simulink model "allModes2"  (R2019a)
settings: Solver=FixedStepAuto  StartTime=0.0  StopTime=inf  FixedStep=1/1000  RelTol=1e-3  EnableMultiTasking=on
undefined symbols (not defined in the file or in its folder): A0, A1, D0, D1, D10, D11, D12, D13, D2, D3, D4, D5, D6, D7, D8, D9, PTA0, PTA1, PTA2, PTB2, PTB23, PTB3, PTB9, PTC16, PTC17, PTC2, PTC3, PTC4, PTD0, PTD1, PTD2, PTD3
libraries: frdmk64flib x22, etargetslib x21, dspstat3 x2
settings Model: SimulationMode=accelerator  ExtModeTrigDuration=5  OrderedModelArguments=off  Creator=adrso  LastModifiedBy=abhis
settings OptimizationCC: EnhancedBackFolding=on  PassReuseOutputArgsAs=Individual arguments  MaxStackSize=64  OptimizeBlockOrder=speed  DifferentSizesBufferReuse=on  OptimizationCustomize=off
settings DebuggingCC: ParameterTunabilityLossMsg=error
settings HardwareCC: ProdBitPerPointer=32  ProdBitPerSizeT=32  ProdBitPerPtrDiffT=32  ProdLargestAtomicInteger=Long  ProdLargestAtomicFloat=Double  ProdWordSize=32  ProdHWDeviceType=ARM Compatible->ARM Cortex
settings SFSimCC: MATLABDynamicMemAlloc=off
settings RTWCC: SystemTargetFile=ert.tlc  HardwareBoard=NXP FRDM-K64F  TLCOptions="-aInlineSetEventsForThisBaseRateFcn=TLC_FALSE -aSuppressMultiTaskScheduler=TLC_FALSE  -aRateBasedStepFcn=0"  TemplateMakefile=ert_default_tmf  GenerateReport=on  Toolchain=GNU Tools for ARM Embedded Processors  BuildConfiguration=Faster Runs  IncludeHyperlinkInReport=on  LaunchReport=on  GenerateTraceInfo=on  GenerateTraceReport=on  GenerateTraceReportSl=on  GenerateTraceReportSf=on  GenerateTraceReportEml=on
settings CodeAppCC: ForceParamTrailComments=on  IgnoreCustomStorageClasses=off  OperatorAnnotations=on  SimulinkDataObjDesc=on  SFDataObjDesc=on  InsertBlockDesc=on
settings ERTTargetCC: SupportContinuousTime=on

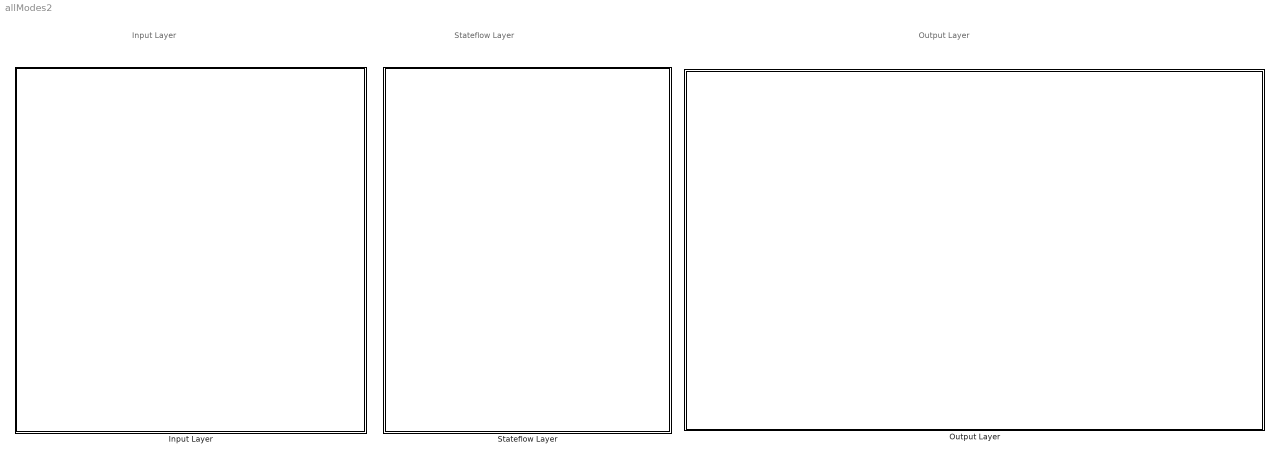
== system allModes2 ==
  note: Input Layer
  note: Stateflow Layer
  note: Output Layer
  Input Layer : Subsystem
      mask Display: image('pacemakerInChest.jpg');
  Output Layer : Subsystem
      mask Display: image('frdmk64f.jpg');
  Stateflow Layer : Subsystem
      mask Display: image('matlabMeme.png');

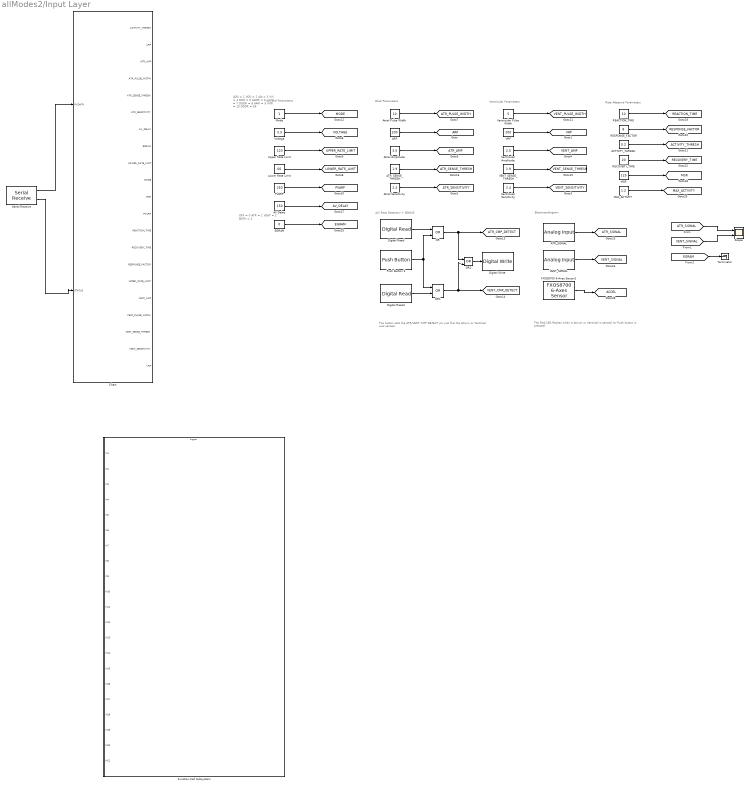
== system allModes2/Input Layer ==
  note: Electrocardiogram
  note: Rate Adaptive Parameters
  note: AOO = 1
      | VOO = 2
      | AAI = 3
      | VVI = 4
      | DOO = 5
      | AOOR = 6
      | VOOR = 7
      | DOOR = 8
      | AAIR = 9
      | VVIR = 10
      | DDDR = 69
  note: The Red LED flashes when a Atrium or Ventrical
      | is sensed (or Push button is pressed)
  note: The button sets the ATR/VENT CMP DETECT
      | pin just like the Atrium or Ventrical was sensed
  note: Ventricular Parameters
  note: Atrial Parameters
  note: A/V Pace Detection + BONUS
  note: General Parameters
  note: OFF = 0
      | ATR = 1
      | VENT = 2
      | BOTH = 3
  ACTIVITY_THRESH : Constant  Value=0.2  OutDataTypeStr=double
  ARP : Constant  Value=200  OutDataTypeStr=uint16
  ATR_SENSE_THRESH : Constant  Value=1.9  OutDataTypeStr=double
  ATR_SIGNAL : frdmk64flib/Analog Input  Whichpin=PTB2 (A0)  SampleTime=-1
      settings: SourceProductName=Simulink Coder Support Package for NXP FRDM-K64F Board
  AV Delay : Constant  Value=150  OutDataTypeStr=uint16
  Atrial Amplitude : Constant  Value=3.5  OutDataTypeStr=double
  Atrial Pulse Width : Constant  Value=10  OutDataTypeStr=uint16
  Atrial Sensitivity : Constant  Value=2.4  OutDataTypeStr=double
  Chart : Stateflow chart  BlockKeywords=__PRM__SERIALIZED__DATA__:Stateflow Chart,Stateflow Diagram  TreatAsAtomicUnit=on
  Digital Read : frdmk64flib/Digital Read  Whichpin=PTC16 (D0)  SampleTime=-1
      settings: SourceProductName=Simulink Coder Support Package for NXP FRDM-K64F Board
  Digital Read1 : frdmk64flib/Digital Read  Whichpin=PTC17 (D1)  SampleTime=-1
      settings: SourceProductName=Simulink Coder Support Package for NXP FRDM-K64F Board
  Digital Write : frdmk64flib/Digital Write  Whichpin=RED_LED
      settings: SourceProductName=Simulink Coder Support Package for NXP FRDM-K64F Board
  EGRAM : Constant  Value=0  OutDataTypeStr=uint16
  FXOS8700 6-Axes Sensor1 : frdmk64flib/FXOS8700 6-Axes Sensor  Activesensor=Accelerometer only  ODR=100Hz  HybridODR=400Hz  Accelfullrange=-4g to +4g  SampleTime=1/100
      settings: SourceProductName=Simulink Coder Support Package for NXP FRDM-K64F Board
  Function-Call Subsystem : Subsystem  TreatAsAtomicUnit=on
  Lower Rate Limit : Constant  Value=60  OutDataTypeStr=uint16
  MAX_ACTIVITY : Constant  Value=1.2  OutDataTypeStr=double
  MSR : Constant  Value=125  OutDataTypeStr=uint16
  Mode : Constant  OutDataTypeStr=uint8
  OR : Logic  Operator=OR  IconShape=distinctive  AllPortsSameDT=off  OutDataTypeStr=boolean
  OR1 : Logic  Operator=OR  IconShape=distinctive  AllPortsSameDT=off  OutDataTypeStr=boolean
  OR2 : Logic  Operator=OR  IconShape=distinctive  AllPortsSameDT=off  OutDataTypeStr=boolean
  PVARP : Constant  Value=250  OutDataTypeStr=uint16
  Push Button 3 : frdmk64flib/Push Button  Whichswitch=SW3  SampleTime1=-1
      settings: SourceProductName=Simulink Coder Support Package for NXP FRDM-K64F Board
  "REACTION_TIME " : Constant  Value=10  OutDataTypeStr=uint16
  RECOVERY_TIME : Constant  Value=20  OutDataTypeStr=uint16
  RESPONSE_FACTOR : Constant  Value=8  OutDataTypeStr=uint16
  Scope : Scope  NumInputPorts=2
  Serial Receive : frdmk64flib/Serial Receive  SCIModule=0  Baudrate=uint32(9600)  Parity=None  StopBits=1  HardwareFlowControl=None  ByteOrder=LittleEndian  DataType=uint8  DataLength=87  BlockingMode=off  OutputStatus=on  SampleTime=-1
      settings: SourceProductName=Simulink Coder Support Package for NXP FRDM-K64F Board
  Terminator : Terminator
  Upper Rate Limit : Constant  Value=120  OutDataTypeStr=uint16
  VENT_SENSE_THRESH : Constant  Value=1.9  OutDataTypeStr=double
  VENT_SIGNAL : frdmk64flib/Analog Input  Whichpin=PTB3 (A1)  SampleTime=-1
      settings: SourceProductName=Simulink Coder Support Package for NXP FRDM-K64F Board
  VRP : Constant  Value=200  OutDataTypeStr=uint16
  Ventricular Amplitude : Constant  Value=2.5  OutDataTypeStr=double
  Ventricular Pulse Width : Constant  Value=5  OutDataTypeStr=uint16
  Ventricular Sensitivity : Constant  Value=2.4  OutDataTypeStr=double
  Voltage : Constant  Value=3.3  OutDataTypeStr=double
  tag scope: ACCEL=global, ACTIVITY_THRESH=global, ARP=global, ATR_AMP=global, ATR_CMP_DETECT=global, ATR_PULSE_WIDTH=global, ATR_SENSE_THRESH=global, ATR_SENSITIVITY=global, ATR_SIGNAL=global, AV_DELAY=global, EGRAM=global, LOWER_RATE_LIMIT=global, MAX_ACTIVITY=global, MODE=global, MSR=global, PVARP=global, REACTION_TIME=global, RECOVERY_TIME=global, RESPONSE_FACTOR=global, UPPER_RATE_LIMIT=global, VENT_AMP=global, VENT_CMP_DETECT=global, VENT_PULSE_WIDTH=global, VENT_SENSE_THRESH=global, VENT_SENSITIVITY=global, VENT_SIGNAL=global, VOLTAGE=global, VRP=global
  wires:
  Ventricular Amplitude/1 -> [VENT_AMP]
  ARP/1 -> [ARP]
  Atrial Amplitude/1 -> [ATR_AMP]
  VRP/1 -> [VRP]
  Voltage/1 -> [VOLTAGE]
  Atrial Sensitivity/1 -> [ATR_SENSITIVITY]
  Ventricular Sensitivity/1 -> [VENT_SENSITIVITY]
  Upper Rate Limit/1 -> [UPPER_RATE_LIMIT]
  Mode/1 -> [MODE]
  Lower Rate Limit/1 -> [LOWER_RATE_LIMIT]
  Ventricular Pulse Width/1 -> [VENT_PULSE_WIDTH]
  Atrial Pulse Width/1 -> [ATR_PULSE_WIDTH]
  Digital Read1/1 -> OR1/2
  VENT_SENSE_THRESH/1 -> [VENT_SENSE_THRESH]
  ATR_SENSE_THRESH/1 -> [ATR_SENSE_THRESH]
  OR/1 -> OR2/1, [ATR_CMP_DETECT]
  Digital Read/1 -> OR/1
  Push Button 3/1 -> OR/2, OR1/1
  OR1/1 -> OR2/2, [VENT_CMP_DETECT]
  OR2/1 -> Digital Write/1
  PVARP/1 -> [PVARP]
  AV Delay/1 -> [AV_DELAY]
  "REACTION_TIME "/1 -> [REACTION_TIME]
  RESPONSE_FACTOR/1 -> [RESPONSE_FACTOR]
  ACTIVITY_THRESH/1 -> [ACTIVITY_THRESH]
  RECOVERY_TIME/1 -> [RECOVERY_TIME]
  MSR/1 -> [MSR]
  ATR_SIGNAL/1 -> [ATR_SIGNAL]
  VENT_SIGNAL/1 -> [VENT_SIGNAL]
  [VENT_SIGNAL] -> Scope/2
  [ATR_SIGNAL] -> Scope/1
  EGRAM/1 -> [EGRAM]
  [EGRAM] -> Terminator/1
  MAX_ACTIVITY/1 -> [MAX_ACTIVITY]
  FXOS8700 6-Axes Sensor1/1 -> [ACCEL]
  Serial Receive/2 -> Chart/2(STATUS)
  Serial Receive/1 -> Chart/1(RXDATA)

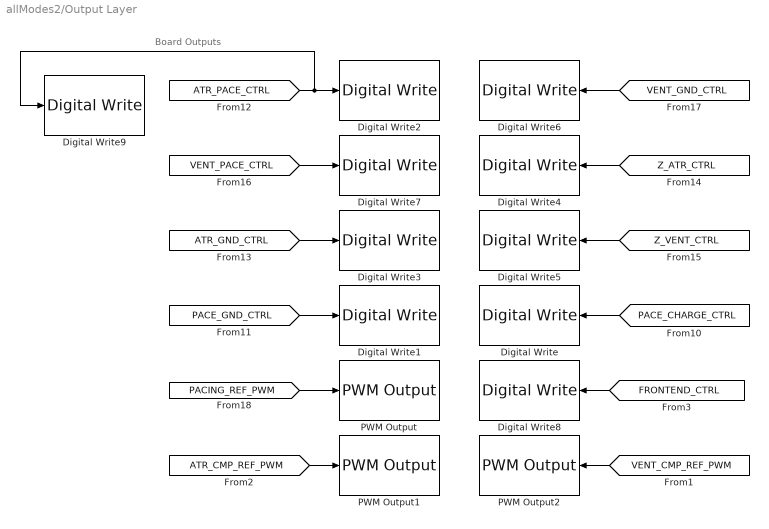
== system allModes2/Output Layer ==
  note: Board Outputs
  Digital Write : frdmk64flib/Digital Write  Whichpin=PTB9 (D2)
      settings: SourceProductName=Simulink Coder Support Package for NXP FRDM-K64F Board
  Digital Write1 : frdmk64flib/Digital Write  Whichpin=PTD0 (D10)
      settings: SourceProductName=Simulink Coder Support Package for NXP FRDM-K64F Board
  Digital Write2 : frdmk64flib/Digital Write  Whichpin=PTA0 (D8)
      settings: SourceProductName=Simulink Coder Support Package for NXP FRDM-K64F Board
  Digital Write3 : frdmk64flib/Digital Write  Whichpin=PTD2 (D11)
      settings: SourceProductName=Simulink Coder Support Package for NXP FRDM-K64F Board
  Digital Write4 : frdmk64flib/Digital Write  Whichpin=PTB23 (D4)
      settings: SourceProductName=Simulink Coder Support Package for NXP FRDM-K64F Board
  Digital Write5 : frdmk64flib/Digital Write  Whichpin=PTC3 (D7)
      settings: SourceProductName=Simulink Coder Support Package for NXP FRDM-K64F Board
  Digital Write6 : frdmk64flib/Digital Write  Whichpin=PTD3 (D12)
      settings: SourceProductName=Simulink Coder Support Package for NXP FRDM-K64F Board
  Digital Write7 : frdmk64flib/Digital Write  Whichpin=PTC4 (D9)
      settings: SourceProductName=Simulink Coder Support Package for NXP FRDM-K64F Board
  Digital Write8 : frdmk64flib/Digital Write  Whichpin=PTD1 (D13)
      settings: SourceProductName=Simulink Coder Support Package for NXP FRDM-K64F Board
  Digital Write9 : frdmk64flib/Digital Write  Whichpin=GREEN_LED
      settings: SourceProductName=Simulink Coder Support Package for NXP FRDM-K64F Board
  PWM Output : frdmk64flib/PWM Output  Whichpin=PTA2 (D5)  InitialFrequency=2000  InitialDutyCycle=30
      settings: SourceProductName=Simulink Coder Support Package for NXP FRDM-K64F Board
  PWM Output1 : frdmk64flib/PWM Output  Whichpin=PTC2 (D6)  InitialFrequency=2000  InitialDutyCycle=30
      settings: SourceProductName=Simulink Coder Support Package for NXP FRDM-K64F Board
  PWM Output2 : frdmk64flib/PWM Output  Whichpin=PTA1 (D3)  InitialFrequency=2000  InitialDutyCycle=30
      settings: SourceProductName=Simulink Coder Support Package for NXP FRDM-K64F Board
  wires:
  [PACING_REF_PWM] -> PWM Output/1
  [VENT_GND_CTRL] -> Digital Write6/1
  [ATR_GND_CTRL] -> Digital Write3/1
  [VENT_PACE_CTRL] -> Digital Write7/1
  [PACE_CHARGE_CTRL] -> Digital Write/1
  [ATR_PACE_CTRL] -> Digital Write9/1, Digital Write2/1
  [Z_VENT_CTRL] -> Digital Write5/1
  [Z_ATR_CTRL] -> Digital Write4/1
  [PACE_GND_CTRL] -> Digital Write1/1
  [ATR_CMP_REF_PWM] -> PWM Output1/1
  [VENT_CMP_REF_PWM] -> PWM Output2/1
  [FRONTEND_CTRL] -> Digital Write8/1

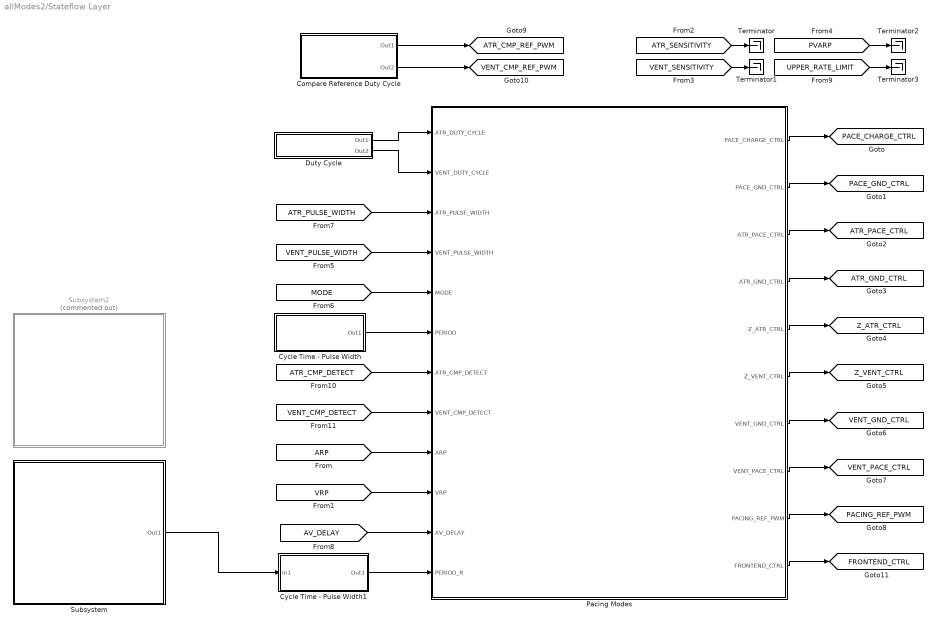
== system allModes2/Stateflow Layer ==
  Compare Reference Duty Cycle : Subsystem
  Cycle Time - Pulse Width : Subsystem
  Cycle Time - Pulse Width1 : Subsystem
  Duty Cycle : Subsystem
  Pacing Modes : Stateflow chart  BlockKeywords=__PRM__SERIALIZED__DATA__:Stateflow Chart,Stateflow Diagram  TreatAsAtomicUnit=on
  Subsystem : Subsystem
  Subsystem2 : Subsystem  Commented=on
  Terminator{,1..3} (4 alike) : Terminator
  tag scope: ATR_CMP_REF_PWM=global, ATR_GND_CTRL=global, ATR_PACE_CTRL=global, FRONTEND_CTRL=global, PACE_CHARGE_CTRL=global, PACE_GND_CTRL=global, PACING_REF_PWM=global, VENT_CMP_REF_PWM=global, VENT_GND_CTRL=global, VENT_PACE_CTRL=global, Z_ATR_CTRL=global, Z_VENT_CTRL=global
  wires:
  [ATR_PULSE_WIDTH] -> Pacing Modes/3(ATR_PULSE_WIDTH)
  [VENT_PULSE_WIDTH] -> Pacing Modes/4(VENT_PULSE_WIDTH)
  Duty Cycle/1(Out1) -> Pacing Modes/1(ATR_DUTY_CYCLE)
  Duty Cycle/2(Out2) -> Pacing Modes/2(VENT_DUTY_CYCLE)
  Pacing Modes/6(Z_VENT_CTRL) -> [Z_VENT_CTRL]
  Pacing Modes/8(VENT_PACE_CTRL) -> [VENT_PACE_CTRL]
  Pacing Modes/4(ATR_GND_CTRL) -> [ATR_GND_CTRL]
  Pacing Modes/3(ATR_PACE_CTRL) -> [ATR_PACE_CTRL]
  Pacing Modes/9(PACING_REF_PWM) -> [PACING_REF_PWM]
  Pacing Modes/2(PACE_GND_CTRL) -> [PACE_GND_CTRL]
  Pacing Modes/1(PACE_CHARGE_CTRL) -> [PACE_CHARGE_CTRL]
  Pacing Modes/5(Z_ATR_CTRL) -> [Z_ATR_CTRL]
  Pacing Modes/7(VENT_GND_CTRL) -> [VENT_GND_CTRL]
  [MODE] -> Pacing Modes/5(MODE)
  Cycle Time - Pulse Width/1(Out1) -> Pacing Modes/6(PERIOD)
  [VENT_CMP_DETECT] -> Pacing Modes/8(VENT_CMP_DETECT)
  [ATR_CMP_DETECT] -> Pacing Modes/7(ATR_CMP_DETECT)
  Pacing Modes/10(FRONTEND_CTRL) -> [FRONTEND_CTRL]
  [ARP] -> Pacing Modes/9(ARP)
  [VRP] -> Pacing Modes/10(VRP)
  Compare Reference Duty Cycle/1(Out1) -> [ATR_CMP_REF_PWM]
  Compare Reference Duty Cycle/2(Out2) -> [VENT_CMP_REF_PWM]
  [ATR_SENSITIVITY] -> Terminator/1
  [VENT_SENSITIVITY] -> Terminator1/1
  [UPPER_RATE_LIMIT] -> Terminator3/1
  [PVARP] -> Terminator2/1
  [AV_DELAY] -> Pacing Modes/11(AV_DELAY)
  Cycle Time - Pulse Width1/1(Out1) -> Pacing Modes/12(PERIOD_R)
  Subsystem/1(Out1) -> Cycle Time - Pulse Width1/1(In1)

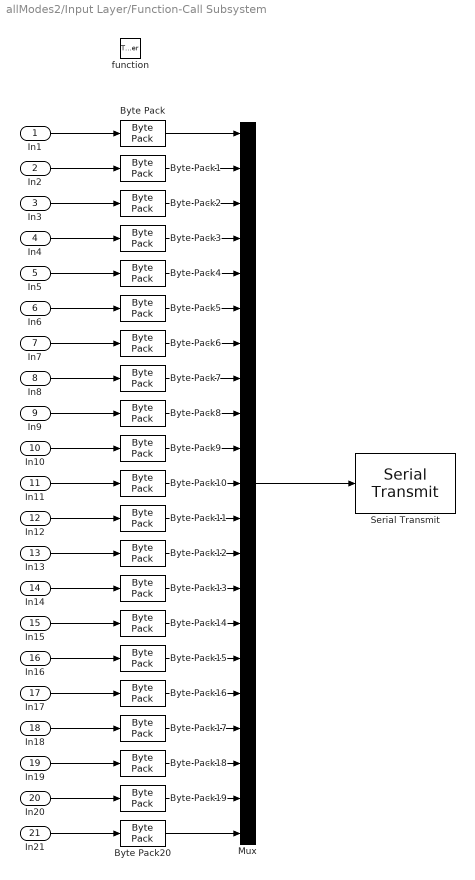
== system allModes2/Input Layer/Function-Call Subsystem ==
  In1 : Inport
  In2 : Inport  Port=2
  In3 : Inport  Port=3
  In4 : Inport  Port=4
  In5 : Inport  Port=5
  In6 : Inport  Port=6
  In7 : Inport  Port=7
  In8 : Inport  Port=8
  In9 : Inport  Port=9
  In10 : Inport  Port=10
  In11 : Inport  Port=11
  In12 : Inport  Port=12
  In13 : Inport  Port=13
  In14 : Inport  Port=14
  In15 : Inport  Port=15
  In16 : Inport  Port=16
  In17 : Inport  Port=17
  In18 : Inport  Port=18
  In19 : Inport  Port=19
  In20 : Inport  Port=20
  In21 : Inport  Port=21
  function : TriggerPort  TriggerType=function-call  IsSimulinkFunction=on  FunctionName=SEND_PARAMETERS  VariantControl=Variant
  Byte Pack{,1..20} (21 alike) : etargetslib/Byte Pack  datatypes={'double'}  byteAlign=1
      settings: SourceProductName=MATLAB Coder
  Mux : Mux  Inputs=21
  Serial Transmit : frdmk64flib/Serial Transmit  SCIModule=0  Baudrate=uint32(9600)  Parity=None  StopBits=1  HardwareFlowControl=None  ByteOrder=LittleEndian  BlockingMode=on  OutputStatus=off
      settings: SourceProductName=Simulink Coder Support Package for NXP FRDM-K64F Board
  wires:
  In1/1 -> Byte Pack/1
  In2/1 -> Byte Pack1/1
  In3/1 -> Byte Pack2/1
  In4/1 -> Byte Pack3/1
  In5/1 -> Byte Pack4/1
  In6/1 -> Byte Pack5/1
  In7/1 -> Byte Pack6/1
  In8/1 -> Byte Pack7/1
  In9/1 -> Byte Pack8/1
  In10/1 -> Byte Pack9/1
  In11/1 -> Byte Pack10/1
  In12/1 -> Byte Pack11/1
  In13/1 -> Byte Pack12/1
  In14/1 -> Byte Pack13/1
  In15/1 -> Byte Pack14/1
  In16/1 -> Byte Pack15/1
  In17/1 -> Byte Pack16/1
  In18/1 -> Byte Pack17/1
  In19/1 -> Byte Pack18/1
  In20/1 -> Byte Pack19/1
  In21/1 -> Byte Pack20/1
  Byte Pack/1 -> Mux/1
  Byte Pack1/1 -> Mux/2
  Byte Pack2/1 -> Mux/3
  Byte Pack3/1 -> Mux/4
  Byte Pack4/1 -> Mux/5
  Byte Pack5/1 -> Mux/6
  Byte Pack6/1 -> Mux/7
  Byte Pack7/1 -> Mux/8
  Byte Pack8/1 -> Mux/9
  Byte Pack9/1 -> Mux/10
  Byte Pack10/1 -> Mux/11
  Byte Pack11/1 -> Mux/12
  Byte Pack12/1 -> Mux/13
  Byte Pack13/1 -> Mux/14
  Byte Pack14/1 -> Mux/15
  Byte Pack15/1 -> Mux/16
  Byte Pack16/1 -> Mux/17
  Byte Pack17/1 -> Mux/18
  Byte Pack18/1 -> Mux/19
  Byte Pack19/1 -> Mux/20
  Byte Pack20/1 -> Mux/21
  Mux/1 -> Serial Transmit/1

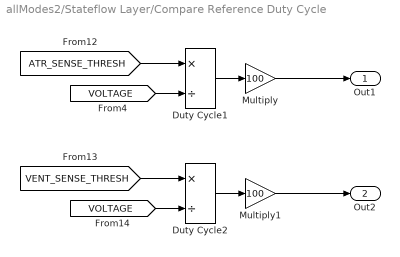
== system allModes2/Stateflow Layer/Compare Reference Duty Cycle ==
  Duty Cycle1 : Product  Inputs=*/
  Duty Cycle2 : Product  Inputs=*/
  Multiply : Gain  Gain=100
  Multiply1 : Gain  Gain=100
  Out1 : Outport
  Out2 : Outport  Port=2
  wires:
  Multiply1/1 -> Out2/1
  [VENT_SENSE_THRESH] -> Duty Cycle2/1
  [VOLTAGE] -> Duty Cycle1/2
  [VOLTAGE] -> Duty Cycle2/2
  Duty Cycle2/1 -> Multiply1/1
  [ATR_SENSE_THRESH] -> Duty Cycle1/1
  Duty Cycle1/1 -> Multiply/1
  Multiply/1 -> Out1/1

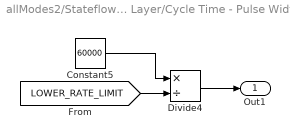
== system allModes2/Stateflow Layer/Cycle Time - Pulse Width ==
  Constant5 : Constant  Value=60000  OutDataTypeStr=uint16
  Divide4 : Product  Inputs=*/  OutDataTypeStr=uint16  RndMeth=Nearest
  Out1 : Outport
  wires:
  [LOWER_RATE_LIMIT] -> Divide4/2
  Constant5/1 -> Divide4/1
  Divide4/1 -> Out1/1

== system allModes2/Stateflow Layer/Cycle Time - Pulse Width1 ==
  In1 : Inport
  Constant5 : Constant  Value=60000  OutDataTypeStr=uint16
  Divide4 : Product  Inputs=*/  OutDataTypeStr=uint16  RndMeth=Nearest
  Out1 : Outport
  wires:
  Constant5/1 -> Divide4/1
  In1/1 -> Divide4/2
  Divide4/1 -> Out1/1

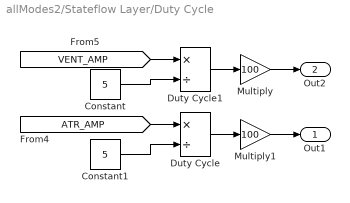
== system allModes2/Stateflow Layer/Duty Cycle ==
  Constant : Constant  Value=5
  Constant1 : Constant  Value=5
  Duty Cycle : Product  Inputs=*/
  Duty Cycle1 : Product  Inputs=*/
  Multiply : Gain  Gain=100
  Multiply1 : Gain  Gain=100
  Out1 : Outport
  Out2 : Outport  Port=2
  wires:
  Constant1/1 -> Duty Cycle/2
  [ATR_AMP] -> Duty Cycle/1
  Constant/1 -> Duty Cycle1/2
  [VENT_AMP] -> Duty Cycle1/1
  Duty Cycle1/1 -> Multiply/1
  Multiply/1 -> Out2/1
  Multiply1/1 -> Out1/1
  Duty Cycle/1 -> Multiply1/1

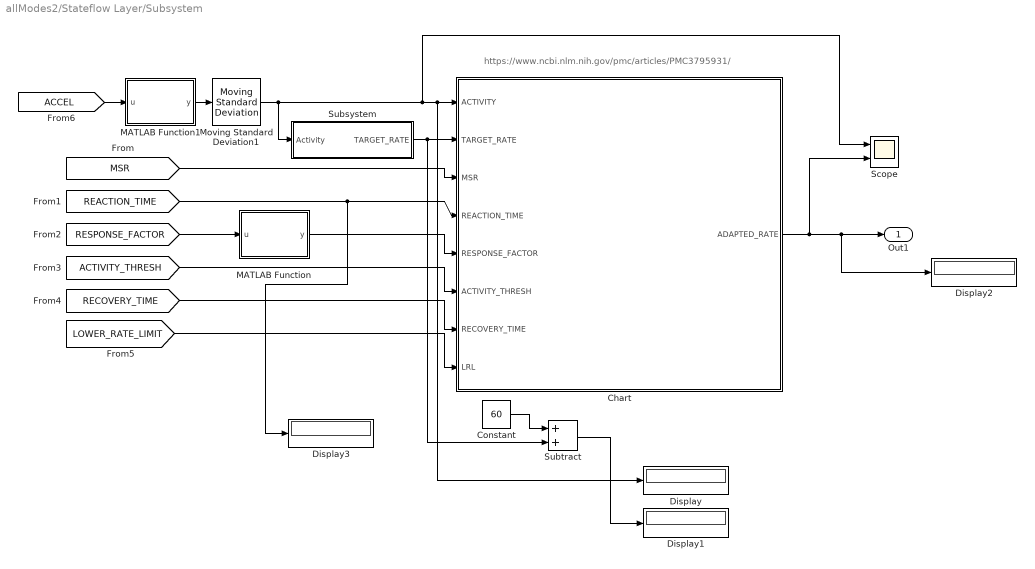
== system allModes2/Stateflow Layer/Subsystem ==
  note: https://www.ncbi.nlm.nih.gov/pmc/articles/PMC3795931/
  Chart : Stateflow chart  BlockKeywords=__PRM__SERIALIZED__DATA__:Stateflow Chart,Stateflow Diagram  TreatAsAtomicUnit=on
  Constant : Constant  Value=60
  Display{,1..3} (4 alike) : Display
  MATLAB Function : MATLAB Function  TreatAsAtomicUnit=on
  MATLAB Function1 : MATLAB Function  TreatAsAtomicUnit=on
  Moving Standard Deviation1 : dspstat3/Moving Standard Deviation  Method=Sliding window  ForgettingFactorPort=off  SpecifyWindowLength=on  WindowLength=64  ForgettingFactor=0.9  SimulateUsing=Code generation
      settings: SourceProductName=DSP System Toolbox  SourceProductBaseCode=DS
  Scope : Scope  NumInputPorts=2
  Subsystem : Subsystem
  Subtract : Sum
  Out1 : Outport
  wires:
  [ACCEL] -> MATLAB Function1/1(u)
  MATLAB Function1/1(y) -> Moving Standard Deviation1/1
  Moving Standard Deviation1/1 -> Scope/1, Display/1, Chart/1(ACTIVITY), Subsystem/1(Activity)
  [MSR] -> Chart/3(MSR)
  [REACTION_TIME] -> Display3/1, Chart/4(REACTION_TIME)
  [ACTIVITY_THRESH] -> Chart/6(ACTIVITY_THRESH)
  [RECOVERY_TIME] -> Chart/7(RECOVERY_TIME)
  [LOWER_RATE_LIMIT] -> Chart/8(LRL)
  Subsystem/1(TARGET_RATE) -> Subtract/2, Chart/2(TARGET_RATE)
  [RESPONSE_FACTOR] -> MATLAB Function/1(u)
  MATLAB Function/1(y) -> Chart/5(RESPONSE_FACTOR)
  Chart/1(ADAPTED_RATE) -> Display2/1, Out1/1, Scope/2
  Constant/1 -> Subtract/1
  Subtract/1 -> Display1/1

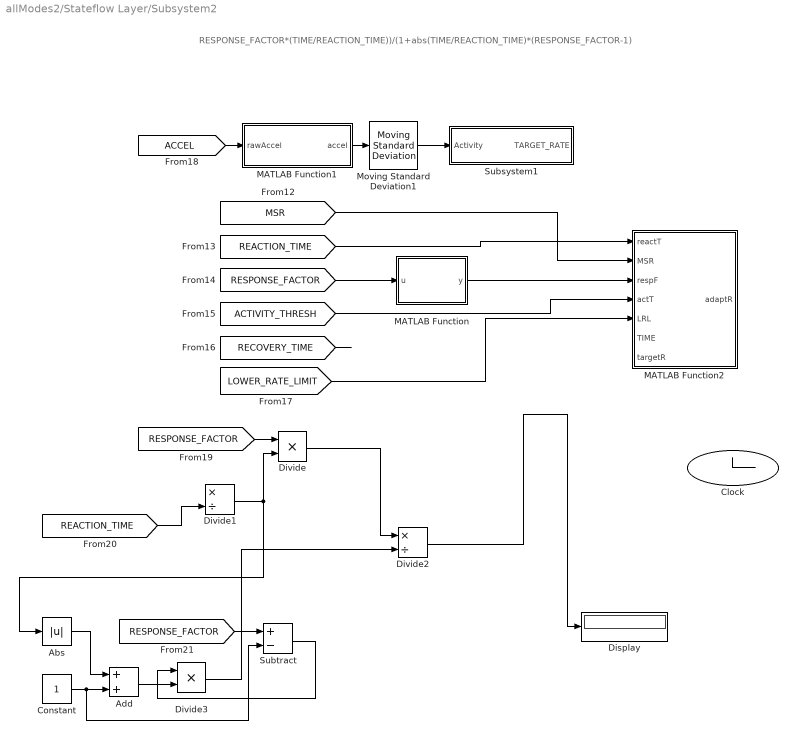
== system allModes2/Stateflow Layer/Subsystem2 ==
  note: RESPONSE_FACTOR*(TIME/REACTION_TIME))/(1+abs(TIME/REACTION_TIME)*(RESPONSE_FACTOR-1)
  Abs : Abs
  Add : Sum
  Clock : Clock
      settings: Decimation=1000
  Constant : Constant
  Display : Display
  Divide : Product  Inputs=**
  Divide1 : Product  Inputs=*/
  Divide2 : Product  Inputs=*/
  Divide3 : Product  Inputs=**
  MATLAB Function : MATLAB Function  TreatAsAtomicUnit=on
  MATLAB Function1 : MATLAB Function  TreatAsAtomicUnit=on
  MATLAB Function2 : MATLAB Function  TreatAsAtomicUnit=on
  Moving Standard Deviation1 : dspstat3/Moving Standard Deviation  Method=Sliding window  ForgettingFactorPort=off  SpecifyWindowLength=on  WindowLength=600  ForgettingFactor=0.9  SimulateUsing=Code generation
      settings: SourceProductName=DSP System Toolbox  SourceProductBaseCode=DS
  Subsystem1 : Subsystem
  Subtract : Sum  Inputs=+-
  wires:
  Divide2/1 -> Display/1
  [RESPONSE_FACTOR] -> Divide/1
  [RESPONSE_FACTOR] -> Subtract/1
  Abs/1 -> Add/1
  Constant/1 -> Subtract/2, Add/2
  Add/1 -> Divide3/2
  Moving Standard Deviation1/1 -> Subsystem1/1(Activity)
  Divide/1 -> Divide2/1
  ? -> Divide1/1
  [RESPONSE_FACTOR] -> MATLAB Function/1(u)
  MATLAB Function1/1(accel) -> Moving Standard Deviation1/1
  [REACTION_TIME] -> Divide1/2
  [ACCEL] -> MATLAB Function1/1(rawAccel)
  Subtract/1 -> Divide3/1
  Divide1/1 -> Abs/1, Divide/2
  Divide3/1 -> Divide2/2
  MATLAB Function/1(y) -> MATLAB Function2/3(respF)
  [REACTION_TIME] -> MATLAB Function2/1(reactT)
  [MSR] -> MATLAB Function2/2(MSR)
  [ACTIVITY_THRESH] -> MATLAB Function2/4(actT)
  [LOWER_RATE_LIMIT] -> MATLAB Function2/5(LRL)
  [RECOVERY_TIME] -> ?

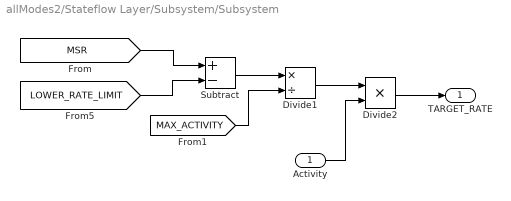
== system allModes2/Stateflow Layer/Subsystem/Subsystem ==
  Activity : Inport
  Divide1 : Product  Inputs=*/
  Divide2 : Product  Inputs=**  OutDataTypeStr=uint16  RndMeth=Nearest
  Subtract : Sum  Inputs=+-
  TARGET_RATE : Outport
  wires:
  [MSR] -> Subtract/1
  [LOWER_RATE_LIMIT] -> Subtract/2
  Subtract/1 -> Divide1/1
  Divide1/1 -> Divide2/1
  Activity/1 -> Divide2/2
  Divide2/1 -> TARGET_RATE/1
  [MAX_ACTIVITY] -> Divide1/2

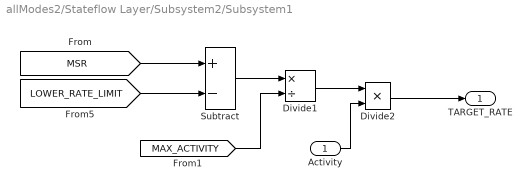
== system allModes2/Stateflow Layer/Subsystem2/Subsystem1 ==
  Activity : Inport
  Divide1 : Product  Inputs=*/
  Divide2 : Product  Inputs=**  OutDataTypeStr=uint16
  Subtract : Sum  Inputs=+-
  TARGET_RATE : Outport
  wires:
  [MSR] -> Subtract/1
  [LOWER_RATE_LIMIT] -> Subtract/2
  Subtract/1 -> Divide1/1
  Divide1/1 -> Divide2/1
  Activity/1 -> Divide2/2
  Divide2/1 -> TARGET_RATE/1
  [MAX_ACTIVITY] -> Divide1/2

== matlab function allModes2/Stateflow Layer/Subsystem/MATLAB Function1 ==
  data: u input; y output
function y = fcn(u)
y = sqrt(u(1)^2+u(2)^2+u(3)^2);

== stateflow chart allModes2/Stateflow Layer/Subsystem/Chart ==
  state Up
    entry:
    TIME = 0
    during:
    ADAPTED_RATE = RESPONSE_FACTOR*(TIME/10)/(1+abs(TIME/10)*(RESPONSE_FACTOR-1))*TARGET_RATE + LRL
    TIME = TIME + 1/1000
    exit:
    TIME = 0
  state Max
  state Down
    entry:
    TIME = 0
    DELTA_RATE = ADAPTED_RATE - LRL
    during:
    ADAPTED_RATE = ADAPTED_RATE - (DELTA_RATE/RECOVERY_TIME)*TIME
    TIME = TIME + 1/1000
    exit:
    TIME = 0
  state Start
    entry:
    ADAPTED_RATE = LRL
  state Min
  Up -> Up [order 3] : [TIME >= REACTION_TIME]{TIME = 0}
  Up -> Max [order 1] : [ADAPTED_RATE == MSR]
  Min -> Up : [ACTIVITY >= ACTIVITY_THRESH]
  Max -> Down : [ACTIVITY < ACTIVITY_THRESH]
  Up -> Down [order 2] : [ACTIVITY < ACTIVITY_THRESH]
  Down -> Up [order 3] : [ACTIVITY >= ACTIVITY_THRESH]
  (default) -> Start
  Start -> Down
  Down -> Min [order 1] : [ADAPTED_RATE == LRL]
  Down -> Down [order 2] : [TIME >= RECOVERY_TIME]{TIME = 0}
  data: ACTIVITY input double; TARGET_RATE input; ADAPTED_RATE output uint16; MSR input uint16; REACTION_TIME input uint16; RESPONSE_FACTOR input double; ACTIVITY_THRESH input double; RECOVERY_TIME input uint16; LRL input uint16; DELTA_RATE local uint16; TIME local double

== stateflow chart allModes2/Stateflow Layer/Pacing Modes ==
  state DOO [group]
    state ATR_DISCHARGING
      during:
      %Discharge C22 into ATR
      %Charge C21
      PACE_CHARGE_CTRL = false
      PACE_GND_CTRL = true
      ATR_PACE_CTRL = true
      ATR_GND_CTRL = false
      Z_ATR_CTRL = false
      Z_VENT_CTRL = false
      VENT_GND_CTRL = false
      VENT_PACE_CTRL = false
    state VENT_CHARGING
      during:
      %Charge C22
      ATR_PACE_CTRL = false
      VENT_PACE_CTRL = false
      PACING_REF_PWM = VENT_DUTY_CYCLE
      PACE_CHARGE_CTRL = true
      %Discharge C21
      PACE_GND_CTRL = true
      VENT_PACE_CTRL = false
      Z_ATR_CTRL = false
      Z_VENT_CTRL = false
      ATR_PACE_CTRL = false
      ATR_GND_CTRL = true
      VENT_GND_CTRL = false
    state VENT_DISCHARGING
      during:
      %Discharge C22 into VENT
      %Charge C21
      PACE_CHARGE_CTRL = false
      PACE_GND_CTRL = true
      ATR_PACE_CTRL = false
      ATR_GND_CTRL = false
      Z_ATR_CTRL = false
      Z_VENT_CTRL = false
      VENT_GND_CTRL = false
      VENT_PACE_CTRL = true
    state ATR_CHARGING
      during:
      %Charge C22
      ATR_PACE_CTRL = false
      VENT_PACE_CTRL = false
      PACING_REF_PWM = VENT_DUTY_CYCLE
      PACE_CHARGE_CTRL = true
      %Discharge C21
      PACE_GND_CTRL = true
      VENT_PACE_CTRL = false
      Z_ATR_CTRL = false
      Z_VENT_CTRL = false
      ATR_PACE_CTRL = false
      ATR_GND_CTRL = false
      VENT_GND_CTRL = true
    DOO.ATR_DISCHARGING -> DOO.VENT_CHARGING : after(ATR_PULSE_WIDTH,msec)
    DOO.VENT_CHARGING -> DOO.VENT_DISCHARGING : after(AV_DELAY - ATR_PULSE_WIDTH, msec)
    DOO.ATR_CHARGING -> DOO.ATR_DISCHARGING [order 2] : after(PERIOD - VENT_PULSE_WIDTH - AV_DELAY, msec)
    DOO.VENT_DISCHARGING -> DOO.ATR_CHARGING : after(VENT_PULSE_WIDTH,msec)
  state DOOR [group]
    state ATR_DISCHARGING
      during:
      %Discharge C22 into ATR
      %Charge C21
      PACE_CHARGE_CTRL = false
      PACE_GND_CTRL = true
      ATR_PACE_CTRL = true
      ATR_GND_CTRL = false
      Z_ATR_CTRL = false
      Z_VENT_CTRL = false
      VENT_GND_CTRL = false
      VENT_PACE_CTRL = false
    state VENT_CHARGING
      during:
      %Charge C22
      ATR_PACE_CTRL = false
      VENT_PACE_CTRL = false
      PACING_REF_PWM = VENT_DUTY_CYCLE
      PACE_CHARGE_CTRL = true
      %Discharge C21
      PACE_GND_CTRL = true
      VENT_PACE_CTRL = false
      Z_ATR_CTRL = false
      Z_VENT_CTRL = false
      ATR_PACE_CTRL = false
      ATR_GND_CTRL = true
      VENT_GND_CTRL = false
    state VENT_DISCHARGING
      during:
      %Discharge C22 into VENT
      %Charge C21
      PACE_CHARGE_CTRL = false
      PACE_GND_CTRL = true
      ATR_PACE_CTRL = false
      ATR_GND_CTRL = false
      Z_ATR_CTRL = false
      Z_VENT_CTRL = false
      VENT_GND_CTRL = false
      VENT_PACE_CTRL = true
    state ATR_CHARGING
      during:
      %Charge C22
      ATR_PACE_CTRL = false
      VENT_PACE_CTRL = false
      PACING_REF_PWM = VENT_DUTY_CYCLE
      PACE_CHARGE_CTRL = true
      %Discharge C21
      PACE_GND_CTRL = true
      VENT_PACE_CTRL = false
      Z_ATR_CTRL = false
      Z_VENT_CTRL = false
      ATR_PACE_CTRL = false
      ATR_GND_CTRL = false
      VENT_GND_CTRL = true
    DOOR.ATR_DISCHARGING -> DOOR.VENT_CHARGING : after(ATR_PULSE_WIDTH,msec)
    DOOR.VENT_CHARGING -> DOOR.VENT_DISCHARGING : after(AV_DELAY - ATR_PULSE_WIDTH, msec)
    DOOR.ATR_CHARGING -> DOOR.ATR_DISCHARGING [order 1] : after(PERIOD_R - VENT_PULSE_WIDTH - AV_DELAY, msec)
    DOOR.VENT_DISCHARGING -> DOOR.ATR_CHARGING : after(VENT_PULSE_WIDTH,msec)
  state AAIR [group]
    state INTERMIDIATE
      during:
      %Discharge C21
      PACE_GND_CTRL = true
      VENT_PACE_CTRL = false
      Z_ATR_CTRL = false
      Z_VENT_CTRL = false
      ATR_PACE_CTRL = false
      ATR_GND_CTRL = true
      VENT_GND_CTRL = false
      %Charge C22
      ATR_PACE_CTRL = false
      VENT_PACE_CTRL = false
      PACING_REF_PWM = ATR_DUTY_CYCLE
      PACE_CHARGE_CTRL = true
    state CHARGING
      during:
      %Charge C22
      ATR_PACE_CTRL = false
      VENT_PACE_CTRL = false
      PACING_REF_PWM = ATR_DUTY_CYCLE
      PACE_CHARGE_CTRL = true
      %Discharge C21
      PACE_GND_CTRL = true
      VENT_PACE_CTRL = false
      Z_ATR_CTRL = false
      Z_VENT_CTRL = false
      ATR_PACE_CTRL = false
      ATR_GND_CTRL = true
      VENT_GND_CTRL = false
    state DISCHARGING
      during:
      %Discharge C22 into ATR
      %Charge C21
      PACE_CHARGE_CTRL = false
      PACE_GND_CTRL = true
      ATR_PACE_CTRL = true
      ATR_GND_CTRL = false
      Z_ATR_CTRL = false
      Z_VENT_CTRL = false
      VENT_GND_CTRL = false
      VENT_PACE_CTRL = false
    AAIR.CHARGING -> (junction 431) [order 1] : [ATR_CMP_DETECT == true]
    (junction 431) -> AAIR.INTERMIDIATE : after(ATR_PULSE_WIDTH,msec)
    AAIR.DISCHARGING -> AAIR.INTERMIDIATE : after(ATR_PULSE_WIDTH, msec)
    AAIR.INTERMIDIATE -> AAIR.CHARGING : after(ARP, msec)
    AAIR.CHARGING -> AAIR.DISCHARGING [order 2] : after(PERIOD_R - ARP - ATR_PULSE_WIDTH, msec)
  state Start
  state AAI [group]
    state INTERMIDIATE
      during:
      %Discharge C21
      PACE_GND_CTRL = true
      VENT_PACE_CTRL = false
      Z_ATR_CTRL = false
      Z_VENT_CTRL = false
      ATR_PACE_CTRL = false
      ATR_GND_CTRL = true
      VENT_GND_CTRL = false
      %Charge C22
      ATR_PACE_CTRL = false
      VENT_PACE_CTRL = false
      PACING_REF_PWM = ATR_DUTY_CYCLE
      PACE_CHARGE_CTRL = true
    state CHARGING
      during:
      %Charge C22
      ATR_PACE_CTRL = false
      VENT_PACE_CTRL = false
      PACING_REF_PWM = ATR_DUTY_CYCLE
      PACE_CHARGE_CTRL = true
      %Discharge C21
      PACE_GND_CTRL = true
      VENT_PACE_CTRL = false
      Z_ATR_CTRL = false
      Z_VENT_CTRL = false
      ATR_PACE_CTRL = false
      ATR_GND_CTRL = true
      VENT_GND_CTRL = false
    state DISCHARGING
      during:
      %Discharge C22 into ATR
      %Charge C21
      PACE_CHARGE_CTRL = false
      PACE_GND_CTRL = true
      ATR_PACE_CTRL = true
      ATR_GND_CTRL = false
      Z_ATR_CTRL = false
      Z_VENT_CTRL = false
      VENT_GND_CTRL = false
      VENT_PACE_CTRL = false
    AAI.CHARGING -> (junction 352) [order 1] : [ATR_CMP_DETECT == true]
    (junction 352) -> AAI.INTERMIDIATE : after(ATR_PULSE_WIDTH,msec)
    AAI.DISCHARGING -> AAI.INTERMIDIATE : after(ATR_PULSE_WIDTH, msec)
    AAI.INTERMIDIATE -> AAI.CHARGING : after(ARP, msec)
    AAI.CHARGING -> AAI.DISCHARGING [order 2] : after(PERIOD - ARP - ATR_PULSE_WIDTH, msec)
  state AAI1 [group]
    state CHARGING
      during:
      %Charge C22
      ATR_PACE_CTRL = false
      VENT_PACE_CTRL = false
      PACING_REF_PWM = ATR_DUTY_CYCLE
      PACE_CHARGE_CTRL = true
      %Discharge C21
      PACE_GND_CTRL = true
      VENT_PACE_CTRL = false
      Z_ATR_CTRL = false
      Z_VENT_CTRL = false
      ATR_PACE_CTRL = false
      ATR_GND_CTRL = true
      VENT_GND_CTRL = false
    state DISCHARGING
      during:
      %Discharge C22 into ATR
      %Charge C21
      PACE_CHARGE_CTRL = false
      PACE_GND_CTRL = true
      ATR_PACE_CTRL = true
      ATR_GND_CTRL = false
      Z_ATR_CTRL = false
      Z_VENT_CTRL = false
      VENT_GND_CTRL = false
      VENT_PACE_CTRL = false
    state w
    AAI1.DISCHARGING -> AAI1.CHARGING : after(ATR_PULSE_WIDTH, msec)
    (junction 410) -> AAI1.CHARGING : after(ATR_PULSE_WIDTH, msec)
    w -> (junction 410) [order 1] : [ATR_CMP_DETECT == true]
    AAI1.CHARGING -> w [order 1] : after(ARP, msec)
    w -> AAI1.DISCHARGING [order 2] : after(PERIOD - ARP - ATR_PULSE_WIDTH, msec)
  state AOO [group]
    state CHARGING
      during:
      %Charge C22
      ATR_PACE_CTRL = false
      VENT_PACE_CTRL = false
      PACING_REF_PWM = ATR_DUTY_CYCLE
      PACE_CHARGE_CTRL = true
      %Discharge C21
      PACE_GND_CTRL = true
      VENT_PACE_CTRL = false
      Z_ATR_CTRL = false
      Z_VENT_CTRL = false
      ATR_PACE_CTRL = false
      ATR_GND_CTRL = true
      VENT_GND_CTRL = false
    state DISCHARGING
      during:
      %Discharge C22 into ATR
      %Charge C21
      PACE_CHARGE_CTRL = false
      PACE_GND_CTRL = true
      ATR_PACE_CTRL = true
      ATR_GND_CTRL = false
      Z_ATR_CTRL = false
      Z_VENT_CTRL = false
      VENT_GND_CTRL = false
      VENT_PACE_CTRL = false
    AOO.CHARGING -> AOO.DISCHARGING [order 1] : after(PERIOD - ATR_PULSE_WIDTH, msec)
    AOO.DISCHARGING -> AOO.CHARGING : after(ATR_PULSE_WIDTH,msec)
  state AOOR [group]
    state CHARGING
      during:
      %Charge C22
      ATR_PACE_CTRL = false
      VENT_PACE_CTRL = false
      PACING_REF_PWM = ATR_DUTY_CYCLE
      PACE_CHARGE_CTRL = true
      %Discharge C21
      PACE_GND_CTRL = true
      VENT_PACE_CTRL = false
      Z_ATR_CTRL = false
      Z_VENT_CTRL = false
      ATR_PACE_CTRL = false
      ATR_GND_CTRL = true
      VENT_GND_CTRL = false
    state DISCHARGING
      during:
      %Discharge C22 into ATR
      %Charge C21
      PACE_CHARGE_CTRL = false
      PACE_GND_CTRL = true
      ATR_PACE_CTRL = true
      ATR_GND_CTRL = false
      Z_ATR_CTRL = false
      Z_VENT_CTRL = false
      VENT_GND_CTRL = false
      VENT_PACE_CTRL = false
    AOOR.CHARGING -> AOOR.DISCHARGING [order 1] : after(PERIOD_R - ATR_PULSE_WIDTH, msec)
    AOOR.DISCHARGING -> AOOR.CHARGING : after(ATR_PULSE_WIDTH,msec)
  state VOO [group]
    state DISCHARGING
      during:
      %Discharge C22 into VENT
      %Charge C21
      PACE_CHARGE_CTRL = false
      PACE_GND_CTRL = true
      ATR_PACE_CTRL = false
      ATR_GND_CTRL = false
      Z_ATR_CTRL = false
      Z_VENT_CTRL = false
      VENT_GND_CTRL = false
      VENT_PACE_CTRL = true
    state CHARGING
      during:
      %Charge C22
      ATR_PACE_CTRL = false
      VENT_PACE_CTRL = false
      PACING_REF_PWM = VENT_DUTY_CYCLE
      PACE_CHARGE_CTRL = true
      %Discharge C21
      PACE_GND_CTRL = true
      VENT_PACE_CTRL = false
      Z_ATR_CTRL = false
      Z_VENT_CTRL = false
      ATR_PACE_CTRL = false
      ATR_GND_CTRL = false
      VENT_GND_CTRL = true
    VOO.CHARGING -> VOO.DISCHARGING [order 1] : after(PERIOD - VENT_PULSE_WIDTH,msec)
    VOO.DISCHARGING -> VOO.CHARGING : after(VENT_PULSE_WIDTH,msec)
  state VOOR [group]
    state DISCHARGING
      during:
      %Discharge C22 into VENT
      %Charge C21
      PACE_CHARGE_CTRL = false
      PACE_GND_CTRL = true
      ATR_PACE_CTRL = false
      ATR_GND_CTRL = false
      Z_ATR_CTRL = false
      Z_VENT_CTRL = false
      VENT_GND_CTRL = false
      VENT_PACE_CTRL = true
    state CHARGING
      during:
      %Charge C22
      ATR_PACE_CTRL = false
      VENT_PACE_CTRL = false
      PACING_REF_PWM = VENT_DUTY_CYCLE
      PACE_CHARGE_CTRL = true
      %Discharge C21
      PACE_GND_CTRL = true
      VENT_PACE_CTRL = false
      Z_ATR_CTRL = false
      Z_VENT_CTRL = false
      ATR_PACE_CTRL = false
      ATR_GND_CTRL = false
      VENT_GND_CTRL = true
    VOOR.CHARGING -> VOOR.DISCHARGING [order 1] : after(PERIOD_R - VENT_PULSE_WIDTH,msec)
    VOOR.DISCHARGING -> VOOR.CHARGING : after(VENT_PULSE_WIDTH,msec)
  state VVI [group]
    state INTERMIDIATE
      during:
      %Discharge C21
      PACE_GND_CTRL = true
      VENT_PACE_CTRL = false
      Z_ATR_CTRL = false
      Z_VENT_CTRL = false
      ATR_PACE_CTRL = false
      ATR_GND_CTRL = false
      VENT_GND_CTRL = true
      %Charge C22
      ATR_PACE_CTRL = false
      VENT_PACE_CTRL = false
      PACING_REF_PWM = VENT_DUTY_CYCLE
      PACE_CHARGE_CTRL = true
    state DISCHARGING
      during:
      %Discharge C22 into VENT
      %Charge C21
      PACE_CHARGE_CTRL = false
      PACE_GND_CTRL = true
      ATR_PACE_CTRL = false
      ATR_GND_CTRL = false
      Z_ATR_CTRL = false
      Z_VENT_CTRL = false
      VENT_GND_CTRL = false
      VENT_PACE_CTRL = true
    state CHARGING
      during:
      %Charge C22
      ATR_PACE_CTRL = false
      VENT_PACE_CTRL = false
      PACING_REF_PWM = VENT_DUTY_CYCLE
      PACE_CHARGE_CTRL = true
      %Discharge C21
      PACE_GND_CTRL = true
      VENT_PACE_CTRL = false
      Z_ATR_CTRL = false
      Z_VENT_CTRL = false
      ATR_PACE_CTRL = false
      ATR_GND_CTRL = false
      VENT_GND_CTRL = true
    VVI.CHARGING -> (junction 357) [order 3] : [VENT_CMP_DETECT == true]
    (junction 357) -> VVI.INTERMIDIATE : after(VENT_PULSE_WIDTH, msec)
    VVI.DISCHARGING -> VVI.INTERMIDIATE : after(VENT_PULSE_WIDTH, msec)
    VVI.INTERMIDIATE -> VVI.CHARGING : after(VRP, msec)
    VVI.CHARGING -> VVI.DISCHARGING [order 1] : after(PERIOD - VRP - VENT_PULSE_WIDTH, msec)
  state VVIR [group]
    state INTERMIDIATE
      during:
      %Discharge C21
      PACE_GND_CTRL = true
      VENT_PACE_CTRL = false
      Z_ATR_CTRL = false
      Z_VENT_CTRL = false
      ATR_PACE_CTRL = false
      ATR_GND_CTRL = false
      VENT_GND_CTRL = true
      %Charge C22
      ATR_PACE_CTRL = false
      VENT_PACE_CTRL = false
      PACING_REF_PWM = VENT_DUTY_CYCLE
      PACE_CHARGE_CTRL = true
    state DISCHARGING
      during:
      %Discharge C22 into VENT
      %Charge C21
      PACE_CHARGE_CTRL = false
      PACE_GND_CTRL = true
      ATR_PACE_CTRL = false
      ATR_GND_CTRL = false
      Z_ATR_CTRL = false
      Z_VENT_CTRL = false
      VENT_GND_CTRL = false
      VENT_PACE_CTRL = true
    state CHARGING
      during:
      %Charge C22
      ATR_PACE_CTRL = false
      VENT_PACE_CTRL = false
      PACING_REF_PWM = VENT_DUTY_CYCLE
      PACE_CHARGE_CTRL = true
      %Discharge C21
      PACE_GND_CTRL = true
      VENT_PACE_CTRL = false
      Z_ATR_CTRL = false
      Z_VENT_CTRL = false
      ATR_PACE_CTRL = false
      ATR_GND_CTRL = false
      VENT_GND_CTRL = true
    VVIR.CHARGING -> (junction 448) [order 2] : [VENT_CMP_DETECT == true]
    (junction 448) -> VVIR.INTERMIDIATE : after(VENT_PULSE_WIDTH, msec)
    VVIR.DISCHARGING -> VVIR.INTERMIDIATE : after(VENT_PULSE_WIDTH, msec)
    VVIR.INTERMIDIATE -> VVIR.CHARGING : after(VRP, msec)
    VVIR.CHARGING -> VVIR.DISCHARGING [order 1] : after(PERIOD_R - VRP - VENT_PULSE_WIDTH, msec)
  state DDDR [group]
    state ATR_DISCHARGING
      during:
      %Discharge C22 into ATR
      %Charge C21
      PACE_CHARGE_CTRL = false
      PACE_GND_CTRL = true
      ATR_PACE_CTRL = true
      ATR_GND_CTRL = false
      Z_ATR_CTRL = false
      Z_VENT_CTRL = false
      VENT_GND_CTRL = false
      VENT_PACE_CTRL = false
    state VENT_CHARGING
      during:
      %Charge C22
      ATR_PACE_CTRL = false
      VENT_PACE_CTRL = false
      PACING_REF_PWM = VENT_DUTY_CYCLE
      PACE_CHARGE_CTRL = true
      %Discharge C21
      PACE_GND_CTRL = true
      VENT_PACE_CTRL = false
      Z_ATR_CTRL = false
      Z_VENT_CTRL = false
      ATR_PACE_CTRL = false
      ATR_GND_CTRL = true
      VENT_GND_CTRL = false
    state VENT_DISCHARGING
      during:
      %Discharge C22 into VENT
      %Charge C21
      PACE_CHARGE_CTRL = false
      PACE_GND_CTRL = true
      ATR_PACE_CTRL = false
      ATR_GND_CTRL = false
      Z_ATR_CTRL = false
      Z_VENT_CTRL = false
      VENT_GND_CTRL = false
      VENT_PACE_CTRL = true
    state ATR_CHARGING
      during:
      %Charge C22
      ATR_PACE_CTRL = false
      VENT_PACE_CTRL = false
      PACING_REF_PWM = VENT_DUTY_CYCLE
      PACE_CHARGE_CTRL = true
      %Discharge C21
      PACE_GND_CTRL = true
      VENT_PACE_CTRL = false
      Z_ATR_CTRL = false
      Z_VENT_CTRL = false
      ATR_PACE_CTRL = false
      ATR_GND_CTRL = false
      VENT_GND_CTRL = true
    DDDR.ATR_DISCHARGING -> DDDR.VENT_CHARGING : after(ATR_PULSE_WIDTH,msec)
    DDDR.VENT_CHARGING -> DDDR.VENT_DISCHARGING : after(AV_DELAY - ATR_PULSE_WIDTH, msec)
    DDDR.ATR_CHARGING -> DDDR.ATR_DISCHARGING [order 1] : after(PERIOD - VENT_PULSE_WIDTH - AV_DELAY, msec)
    DDDR.VENT_DISCHARGING -> DDDR.ATR_CHARGING : after(VENT_PULSE_WIDTH,msec)
  DOOR.ATR_CHARGING -> Start [order 2] : [MODE ~= 8]
  DDDR.ATR_CHARGING -> Start [order 2] : [MODE ~= 69]
  Start -> DOOR.ATR_CHARGING [order 5] : [MODE == 8]
  Start -> AAIR.CHARGING [order 4] : [MODE == 9]
  AAIR.CHARGING -> Start [order 3] : [MODE ~= 9]
  Start -> DDDR.ATR_CHARGING [order 2] : [MODE == 69]
  AAI1.CHARGING -> Start [order 2] : [MODE ~= 31]
  Start -> AAI1.CHARGING [order 6] : [MODE == 31]
  DOO.ATR_CHARGING -> Start [order 1] : [MODE ~= 5]
  VOO.CHARGING -> Start [order 2] : [MODE ~= 2]
  AOO.CHARGING -> Start [order 2] : [MODE ~= 1]
  AAI.CHARGING -> Start [order 3] : [MODE ~= 3]
  VVI.CHARGING -> Start [order 2] : [MODE ~= 4]
  Start -> AAI.CHARGING [order 12] : [MODE == 3]
  Start -> DOO.ATR_CHARGING [order 8] : [MODE == 5]
  VVIR.CHARGING -> Start [order 3] : [MODE ~= 10]
  Start -> AOO.CHARGING [order 1] : [MODE == 1]
  AOOR.CHARGING -> Start [order 2] : [MODE ~= 6]
  VOOR.CHARGING -> Start [order 2] : [MODE ~= 7]
  Start -> VVI.CHARGING [order 11] : [MODE == 4]
  Start -> VOO.CHARGING [order 10] : [MODE == 2]
  Start -> VVIR.CHARGING [order 3] : [MODE == 10]
  Start -> AOOR.CHARGING [order 7] : [MODE == 6]
  Start -> VOOR.CHARGING [order 9] : [MODE == 7]
  (default) -> Start
  data: ATR_DUTY_CYCLE input double; VENT_DUTY_CYCLE input double; ATR_PULSE_WIDTH input uint16; PACE_CHARGE_CTRL output boolean; PACE_GND_CTRL output boolean; ATR_PACE_CTRL output boolean; ATR_GND_CTRL output boolean; Z_ATR_CTRL output boolean =false; Z_VENT_CTRL output boolean =false; VENT_GND_CTRL output boolean; VENT_PACE_CTRL output boolean; PACING_REF_PWM output double; VENT_PULSE_WIDTH input uint16; MODE input uint8; PERIOD input uint16; ATR_CMP_DETECT input boolean; VENT_CMP_DETECT input boolean; FRONTEND_CTRL output boolean =true; ARP input uint16; VRP input uint16; AV_DELAY input uint16; PERIOD_R input uint16

== matlab function allModes2/Stateflow Layer/Subsystem/MATLAB Function ==
  data: u input; y output
function y = fcn(u)

slope = [1:1/3:5];

y = slope(u);

== matlab function allModes2/Stateflow Layer/Subsystem2/MATLAB Function2 ==
  data: reactT input; adaptR output; MSR input; respF input; actT input; LRL input; TIME input; targetR input
function adaptR = fcn(reactT, MSR, respF, actT, LRL, TIME, targetR)

adaptR = respF*(TIME/reactT)/(1+ abs(TIME/reactT)*(respF -1))*targetR - LRL;

== matlab function allModes2/Stateflow Layer/Subsystem2/MATLAB Function ==
  data: u input; y output
function y = fcn(u)

slope = 1:1/3:5;

y = slope(u);

== matlab function allModes2/Stateflow Layer/Subsystem2/MATLAB Function1 ==
  data: rawAccel input; accel output
function accel = fcn(rawAccel)
accel = sqrt(rawAccel(1)^2+rawAccel(2)^2+rawAccel(3)^2);

== stateflow chart allModes2/Input Layer/Chart ==
  state SET_PARAMETERS
    entry:
    MODE = typecast(RXDATA(3:4), 'uint16');
    UPPER_RATE_LIMIT = typecast(RXDATA(5:6), 'uint16');
    LOWER_RATE_LIMIT = typecast(RXDATA(7:8), 'uint16');
    PVARP = typecast(RXDATA(9:10), 'uint16');
    AV_DELAY = typecast(RXDATA(11:12), 'uint16');
    EGRAM = typecast(RXDATA(13:14), 'uint16');
    ATR_PULSE_WIDTH = typecast(RXDATA(15:16), 'uint16');
    ARP = typecast(RXDATA(17:18), 'uint16');
    ATR_AMP  = typecast(RXDATA(19:26), 'double');
    ATR_SENSE_THRESH = typecast(RXDATA(27:34), 'double');
    ATR_SENSITIVITY = typecast(RXDATA(35:42), 'double');
    VENT_PULSE_WIDTH = typecast(RXDATA(43:44), 'uint16');
    VRP = typecast(RXDATA(45:46), 'uint16');
    VENT_AMP = typecast(RXDATA(47:54), 'double');
    VENT_SENSE_THRESH = typecast(RXDATA(55:62), 'double');
    VENT_SENSITIVITY = typecast(RXDATA(65:72), 'double');
    REACTION_TIME = typecast(RXDATA(72:73), 'uint16');
    RESPONSE_FACTOR = typecast(RXDATA(74:75), 'uint16');
    ACTIVITY_THRESH = typecast(RXDATA(76:83), 'double');
    RECOVERY_TIME = typecast(RXDATA(84:85), 'uint16');
    MSR = typecast(RXDATA(86:87), 'uint16');
  state INITIAL
    %Setting the initial parameters
    entry:
    MODE = 0;
    UPPER_RATE_LIMIT = 120;
    LOWER_RATE_LIMIT = 60;
    PVARP = 250;
    AV_DELAY = 150;
    EGRAM = 0;
    ATR_PULSE_WIDTH = 10;
    ARP = 200;
    ATR_AMP  = 3.5;
    ATR_SENSE_THRESH = 1.9;
    ATR_SENSITIVITY = 2.4;
    VENT_PULSE_WIDTH = 5;
    VRP = 200;
    VENT_AMP = 2.5;
    VENT_SENSE_THRESH = 1.9;
    VENT_SENSITIVITY = 2.4;
    REACTION_TIME = 10;
    RESPONSE_FACTOR = 8;
    ACTIVITY_THRESH = 0;
    RECOVERY_TIME = 20;
    MSR = 125;
  state STANDBY
  state ECHO_PARAMETERS
    entry:
    SEND_PARAMETERS();
  SET_PARAMETERS -> STANDBY
  (default) -> INITIAL
  (junction 9) -> SET_PARAMETERS [order 1] : [RXDATA(2) == hex2dec('7')]
  (junction 7) -> STANDBY [order 2]
  INITIAL -> STANDBY
  STANDBY -> (junction 7) : [STATUS == 0]
  (junction 7) -> (junction 9) [order 1] : [RXDATA(1) == hex2dec('69')]
  (junction 9) -> ECHO_PARAMETERS [order 2] : [RXDATA(2) == hex2dec('21')]
  ECHO_PARAMETERS -> STANDBY
  data: RXDATA input uint8; STATUS input uint8; ACTIVITY_THRESH output double; ARP output uint16; ATR_AMP output double; ATR_PULSE_WIDTH output uint16; ATR_SENSE_THRESH output double; ATR_SENSITIVITY output double; AV_DELAY output uint16; EGRAM output uint16; LOWER_RATE_LIMIT output uint16; MODE output uint16; MSR output uint16; PVARP output uint16; REACTION_TIME output uint16; RECOVERY_TIME output uint16; RESPONSE_FACTOR output uint16; UPPER_RATE_LIMIT output uint16; VENT_AMP output double; VENT_PULSE_WIDTH output uint16; VENT_SENSE_THRESH output double; VENT_SENSITIVITY output double; VRP output uint16
